simulink model "model9_sin"  (R2020b)
settings: Solver=ode4  StartTime=0.0  StopTime=stopTime  RelTol=1e-3
values from neighbouring files (symbols this model uses):
  freq = 0.1    [start_model_silnik.m]
  regP =     [nastawy.mat]    (also in sisoNastawy.mat)
  regPID =     [nastawy.mat]    (also in sisoNastawy.mat)
undefined symbols (not defined in the file or in its folder): model
settings Model: Creator=Robert  LastModifiedBy=Robert

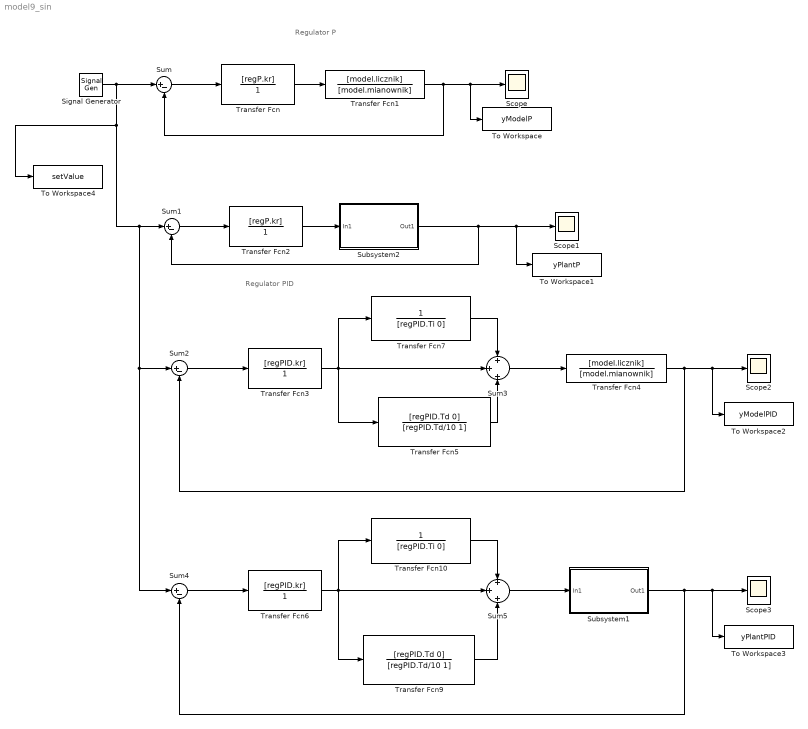
== system model9_sin ==
  note: Regulator P
  note: Regulator PID
  Scope{,1..3} (4 alike) : Scope
  Signal Generator : SignalGenerator  Amplitude=u  Frequency=freq  Units=rad/sec
  Subsystem1 : Subsystem
  Subsystem2 : Subsystem
  Sum{,1..2,4} (4 alike) : Sum  Inputs=|+-
  Sum3 : Sum  Inputs=+|+|+
  Sum5 : Sum  Inputs=+|+|+
  To Workspace : ToWorkspace  VariableName=yModelP  SampleTime=-1
  To Workspace1 : ToWorkspace  VariableName=yPlantP  SampleTime=-1
  To Workspace2 : ToWorkspace  VariableName=yModelPID  SampleTime=-1
  To Workspace3 : ToWorkspace  VariableName=yPlantPID  SampleTime=-1
  To Workspace4 : ToWorkspace  VariableName=setValue  SampleTime=-1
  Transfer Fcn : TransferFcn  Numerator=[regP.kr]  Denominator=[1]
  Transfer Fcn1 : TransferFcn  Numerator=[model.licznik]  Denominator=[model.mianownik]
  Transfer Fcn10 : TransferFcn  Denominator=[regPID.Ti 0]
  Transfer Fcn2 : TransferFcn  Numerator=[regP.kr]  Denominator=[1]
  Transfer Fcn3 : TransferFcn  Numerator=[regPID.kr]  Denominator=[1]
  Transfer Fcn4 : TransferFcn  Numerator=[model.licznik]  Denominator=[model.mianownik]
  Transfer Fcn5 : TransferFcn  Numerator=[regPID.Td 0]  Denominator=[regPID.Td/10 1]
  Transfer Fcn6 : TransferFcn  Numerator=[regPID.kr]  Denominator=[1]
  Transfer Fcn7 : TransferFcn  Denominator=[regPID.Ti 0]
  Transfer Fcn9 : TransferFcn  Numerator=[regPID.Td 0]  Denominator=[regPID.Td/10 1]
  wires:
  Transfer Fcn5/1 -> Sum3/3
  Transfer Fcn6/1 -> Transfer Fcn10/1, Transfer Fcn9/1, Sum5/2
  Sum5/1 -> Subsystem1/1(In1)
  Transfer Fcn9/1 -> Sum5/3
  Sum4/1 -> Transfer Fcn6/1
  Transfer Fcn/1 -> Transfer Fcn1/1
  Subsystem1/1(Out1) -> Sum4/2, Scope3/1, To Workspace3/1
  Transfer Fcn4/1 -> Sum2/2, Scope2/1, To Workspace2/1
  Transfer Fcn10/1 -> Sum5/1
  Transfer Fcn1/1 -> Sum/2, Scope/1, To Workspace/1
  Transfer Fcn7/1 -> Sum3/1
  Transfer Fcn3/1 -> Transfer Fcn5/1, Transfer Fcn7/1, Sum3/2
  Transfer Fcn2/1 -> Subsystem2/1(In1)
  Subsystem2/1(Out1) -> Sum1/2, To Workspace1/1, Scope1/1
  Sum1/1 -> Transfer Fcn2/1
  Sum3/1 -> Transfer Fcn4/1
  Sum2/1 -> Transfer Fcn3/1
  Sum/1 -> Transfer Fcn/1
  Signal Generator/1 -> Sum/1, To Workspace4/1, Sum4/1, Sum2/1, Sum1/1

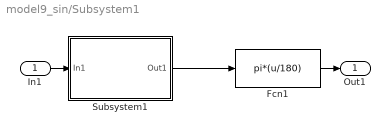
== system model9_sin/Subsystem1 ==
  In1 : Inport
  Fcn1 : Fcn  Expr=pi*(u/180)
  Subsystem1 : Subsystem
  Out1 : Outport
  wires:
  Subsystem1/1(Out1) -> Fcn1/1
  Fcn1/1 -> Out1/1
  In1/1 -> Subsystem1/1(In1)

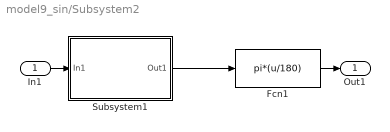
== system model9_sin/Subsystem2 ==
  In1 : Inport
  Fcn1 : Fcn  Expr=pi*(u/180)
  Subsystem1 : Subsystem
  Out1 : Outport
  wires:
  Subsystem1/1(Out1) -> Fcn1/1
  Fcn1/1 -> Out1/1
  In1/1 -> Subsystem1/1(In1)

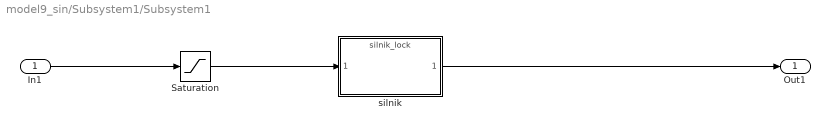
== system model9_sin/Subsystem1/Subsystem1 ==
  In1 : Inport
  Saturation : Saturate  UpperLimit=2  LowerLimit=-2
  silnik : ModelReference  ModelNameDialog=silnik_lock.slxp  ModelReferenceVersion=1.38  CopyOfModelProtected=on
  Out1 : Outport
  wires:
  silnik/1 -> Out1/1
  Saturation/1 -> silnik/1
  In1/1 -> Saturation/1

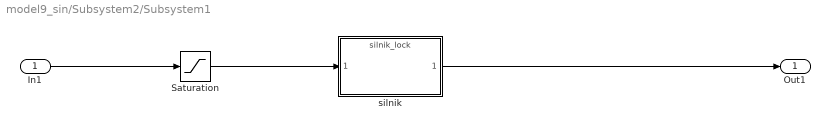
== system model9_sin/Subsystem2/Subsystem1 ==
  In1 : Inport
  Saturation : Saturate  UpperLimit=2  LowerLimit=-2
  silnik : ModelReference  ModelNameDialog=silnik_lock.slxp  ModelReferenceVersion=1.38  CopyOfModelProtected=on
  Out1 : Outport
  wires:
  silnik/1 -> Out1/1
  Saturation/1 -> silnik/1
  In1/1 -> Saturation/1
